simulink model "satellite_dynamics"  (R2016a)
settings: Solver=VariableStepAuto  StartTime=0.0  StopTime=10.0  RelTol=1e-3
values from neighbouring files (symbols this model uses):
  DBG = [MB.m*eye(3) zeros(3,3);zeros(3,3) MB.I]    [exemple_debris.m]    (also in sat_dynamics.m)
  SCtauCGP = [eye(3) -[0 CGPvec(3) -CGPvec(2) ... (first row only)    [exemple_debris.m]    (also in sat_dynamics.m)
undefined symbols (not defined in the file or in its folder): SA
libraries: cstblocks x3
settings Model: Creator=f.sanfedino  LastModifiedBy=f.sanfedino

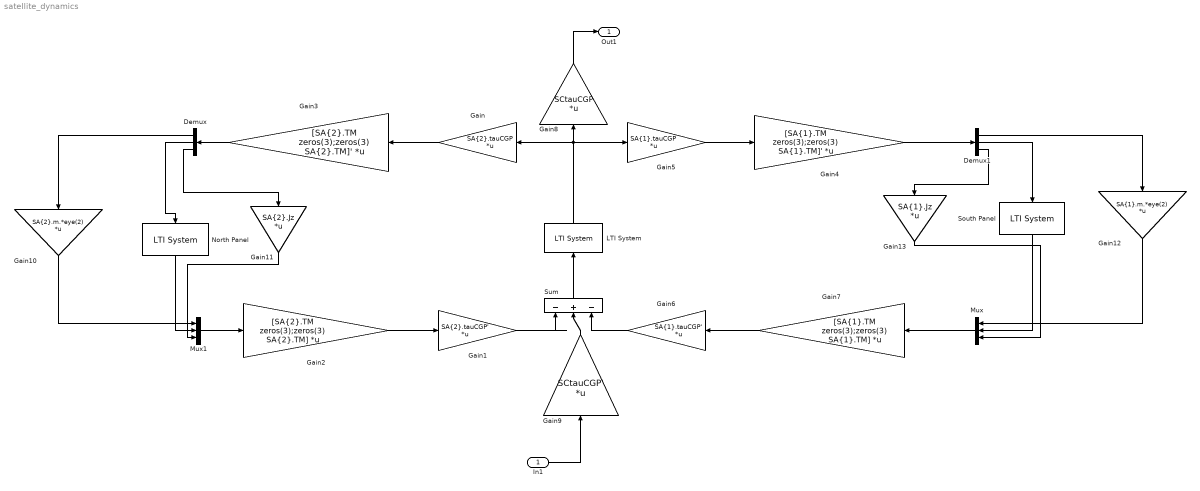
== system satellite_dynamics ==
  In1 : Inport  PortDimensions=6
  Demux : Demux  Outputs=3
  Demux1 : Demux  Outputs=3
  Gain : Gain  Gain=SA{2}.tauCGP  Multiplication=Matrix(K*u)
  Gain1 : Gain  Gain=SA{2}.tauCGP'  Multiplication=Matrix(K*u)
  Gain10 : Gain  Gain=SA{2}.m.*eye(2)  Multiplication=Matrix(K*u)
  Gain11 : Gain  Gain=SA{2}.Jz  Multiplication=Matrix(K*u)
  Gain12 : Gain  Gain=SA{1}.m.*eye(2)  Multiplication=Matrix(K*u)
  Gain13 : Gain  Gain=SA{1}.Jz  Multiplication=Matrix(K*u)
  Gain2 : Gain  Gain=[SA{2}.TM zeros(3);zeros(3) SA{2}.TM]  Multiplication=Matrix(K*u)
  Gain3 : Gain  Gain=[SA{2}.TM zeros(3);zeros(3) SA{2}.TM]'  Multiplication=Matrix(K*u)
  Gain4 : Gain  Gain=[SA{1}.TM zeros(3);zeros(3) SA{1}.TM]'  Multiplication=Matrix(K*u)
  Gain5 : Gain  Gain=SA{1}.tauCGP  Multiplication=Matrix(K*u)
  Gain6 : Gain  Gain=SA{1}.tauCGP'  Multiplication=Matrix(K*u)
  Gain7 : Gain  Gain=[SA{1}.TM zeros(3);zeros(3) SA{1}.TM]  Multiplication=Matrix(K*u)
  Gain8 : Gain  Gain=SCtauCGP  Multiplication=Matrix(K*u)
  Gain9 : Gain  Gain=SCtauCGP'  Multiplication=Matrix(K*u)
  LTI System : cstblocks/LTI System  sys=inv(DBG)  IC=[]
  Mux : Mux  Inputs=3
  Mux1 : Mux  Inputs=3
  North Panel : cstblocks/LTI System  sys=SA{2}.dyn  IC=[]
  South Panel : cstblocks/LTI System  sys=SA{1}.dyn  IC=[]
  Sum : Sum  Inputs=|-+-
  Out1 : Outport
  wires:
  Gain2/1 -> Gain1/1
  Gain/1 -> Gain3/1
  Mux1/1 -> Gain2/1
  LTI System/1 -> Gain/1, Gain8/1, Gain5/1
  Sum/1 -> LTI System/1
  Gain1/1 -> Sum/1
  Gain5/1 -> Gain4/1
  Gain6/1 -> Sum/3
  Gain7/1 -> Gain6/1
  Mux/1 -> Gain7/1
  In1/1 -> Gain9/1
  Gain9/1 -> Sum/2
  Gain8/1 -> Out1/1
  Gain3/1 -> Demux/1
  Demux/1 -> Gain10/1
  Demux/2 -> North Panel/1
  Demux/3 -> Gain11/1
  Gain4/1 -> Demux1/1
  Demux1/1 -> Gain12/1
  Demux1/2 -> South Panel/1
  Demux1/3 -> Gain13/1
  South Panel/1 -> Mux/2
  Gain10/1 -> Mux1/1
  North Panel/1 -> Mux1/2
  Gain11/1 -> Mux1/3
  Gain13/1 -> Mux/3
  Gain12/1 -> Mux/1
